simulink model "CALC_MODEL_FLOAT"  (R2022a)
settings: Solver=VariableStepAuto  StartTime=0.0  StopTime=10.0  RelTol=1e-3
settings Model: Creator=Mykyta  LastModifiedBy=Mykyta

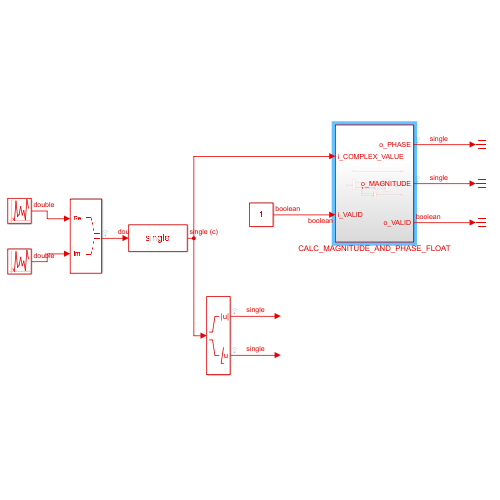
[thumbnail: Simulink's stored preview of the top-level diagram]
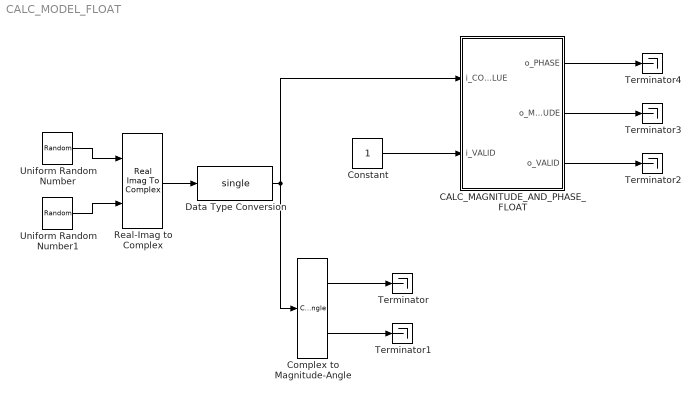
== system CALC_MODEL_FLOAT ==
  CALC_MAGNITUDE_AND_PHASE_FLOAT : Subsystem
  Complex to Magnitude-Angle : ComplexToMagnitudeAngle
  Constant : Constant  OutDataTypeStr=boolean  SampleTime=1
  Data Type Conversion : DataTypeConversion  OutDataTypeStr=single  SaturateOnIntegerOverflow=off  RndMeth=Floor
  Real-Imag to Complex : RealImagToComplex
  Terminator{,1..4} (5 alike) : Terminator
  Uniform Random Number : UniformRandomNumber  Minimum=0  Maximum=16383.999996185302734375  Seed=14  SampleTime=1
  Uniform Random Number1 : UniformRandomNumber  Minimum=0  Maximum=16383.999996185302734375  Seed=15  SampleTime=1
  wires:
  Uniform Random Number/1 -> Real-Imag to Complex/1
  Uniform Random Number1/1 -> Real-Imag to Complex/2
  Complex to Magnitude-Angle/2 -> Terminator1/1
  Complex to Magnitude-Angle/1 -> Terminator/1
  CALC_MAGNITUDE_AND_PHASE_FLOAT/1(o_PHASE) -> Terminator4/1
  CALC_MAGNITUDE_AND_PHASE_FLOAT/2(o_MAGNITUDE) -> Terminator3/1
  Constant/1 -> CALC_MAGNITUDE_AND_PHASE_FLOAT/2(i_VALID)
  CALC_MAGNITUDE_AND_PHASE_FLOAT/3(o_VALID) -> Terminator2/1
  Real-Imag to Complex/1 -> Data Type Conversion/1
  Data Type Conversion/1 -> CALC_MAGNITUDE_AND_PHASE_FLOAT/1(i_COMPLEX_VALUE), Complex to Magnitude-Angle/1

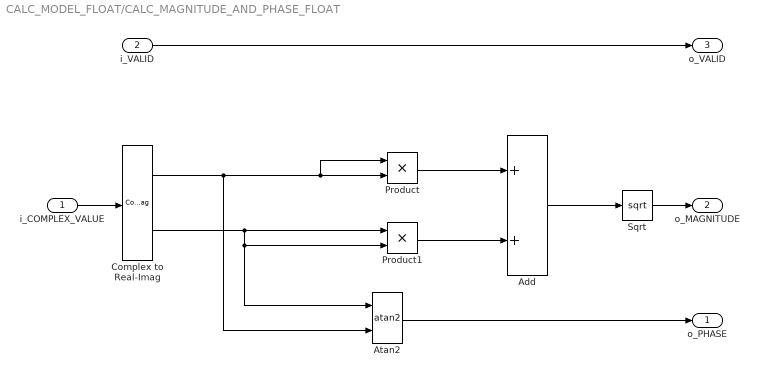
== system CALC_MODEL_FLOAT/CALC_MAGNITUDE_AND_PHASE_FLOAT ==
  i_COMPLEX_VALUE : Inport
  i_VALID : Inport  Port=2  OutDataTypeStr=boolean
  Add : Sum  OutDataTypeStr=single
  Atan2 : Trigonometry  Operator=atan2  NumberOfIterations=20
  Complex to Real-Imag : ComplexToRealImag
  Product : Product  SaturateOnIntegerOverflow=on
  Product1 : Product  LockScale=on
  Sqrt : Sqrt  OutDataTypeStr=single
  o_PHASE : Outport
  o_MAGNITUDE : Outport  Port=2
  o_VALID : Outport  Port=3  OutDataTypeStr=boolean
  wires:
  Complex to Real-Imag/2 -> Product1/1, Atan2/1, Product1/2
  Complex to Real-Imag/1 -> Atan2/2, Product/1, Product/2
  Atan2/1 -> o_PHASE/1
  Product1/1 -> Add/2
  Product/1 -> Add/1
  Add/1 -> Sqrt/1
  Sqrt/1 -> o_MAGNITUDE/1
  i_COMPLEX_VALUE/1 -> Complex to Real-Imag/1
  i_VALID/1 -> o_VALID/1
